simulink model "SYS"  (Simulink 9.2)
settings: Solver=VariableStepAuto  StartTime=0.0  StopTime=10.0  RelTol=1e-3
settings Model: Creator=maman  LastModifiedBy=maman
settings DataIOCC: LimitDataPoints=off  SaveFormat=Dataset  SignalLoggingSaveFormat=Dataset
settings OptimizationCC: LifeSpan=auto
settings DebuggingCC: UnderspecifiedInitializationDetection=Simplified  MergeDetectMultiDrivingBlocksExec=error  FcnCallInpInsideContextMsg=error  StateNameClashWarn=none  SFUnexpectedBacktrackingDiag=error  SFNoUnconditionalDefaultTransitionDiag=error  SFExecutionAtInitializationDiag=warning
settings HardwareCC: ProdBitPerPointer=64  ProdBitPerSizeT=64  ProdBitPerPtrDiffT=64  ProdLargestAtomicFloat=Float  ProdIntDivRoundTo=Zero  ProdEndianess=LittleEndian  ProdWordSize=64  ProdHWDeviceType=Intel->x86-64 (Windows64)
settings ModelReferenceCC: PropagateSignalLabelsOutOfModel=on
settings SFSimCC: SimUseLocalCustomCode=on
settings RTWCC: RTWUseLocalCustomCode=on
settings CodeAppCC: StateflowObjectComments=off
settings GRTTargetCC: TargetLangStandard=C99 (ISO)  GeneratePreprocessorConditionals=Use local settings  CombineOutputUpdateFcns=on  GRTInterface=off
settings ConfigComp: CovMetricSettings=dwe  CovHtmlReporting=off  CovSaveCumulativeToWorkspaceVar=off  CovSaveSingleToWorkspaceVar=off  CovExternalEMLEnable=on

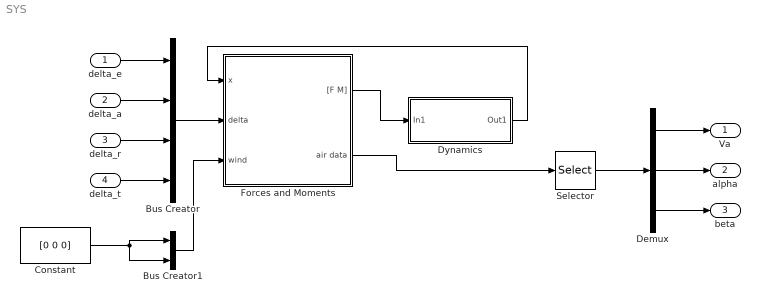
== system SYS ==
  delta_e : Inport
  delta_a : Inport  Port=2
  delta_r : Inport  Port=3
  delta_t : Inport  Port=4
  Bus Creator : BusCreator  Inputs=4
  Bus Creator1 : BusCreator  Inputs=2
  Constant : Constant  Value=[0 0 0]
  Demux : Demux  Outputs=3
  Dynamics : Subsystem  TreatAsAtomicUnit=on
  Forces and Moments : Subsystem  TreatAsAtomicUnit=on
  Selector : Selector  NumberOfDimensions=2  InputPortWidth=3  IndexOptions=Index vector (dialog),Index vector (dialog)  Indices=[1 3],1  OutputSizes=1,1
  Va : Outport
  alpha : Outport  Port=2
  beta : Outport  Port=3
  wires:
  delta_e/1 -> Bus Creator/1
  delta_a/1 -> Bus Creator/2
  delta_r/1 -> Bus Creator/3
  delta_t/1 -> Bus Creator/4
  Bus Creator/1 -> Forces and Moments/2(delta)
  Bus Creator1/1 -> Forces and Moments/3(wind)
  Forces and Moments/1("[F M]") -> Dynamics/1(In1)
  Dynamics/1(Out1) -> Forces and Moments/1(x)
  Forces and Moments/2(air data) -> Selector/1
  Demux/2 -> alpha/1
  Demux/1 -> Va/1
  Demux/3 -> beta/1
  Selector/1 -> Demux/1
  Constant/1 -> Bus Creator1/2, Bus Creator1/1

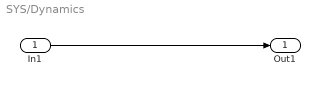
== system SYS/Dynamics ==
  In1 : Inport
  Out1 : Outport
  wires:
  In1/1 -> Out1/1

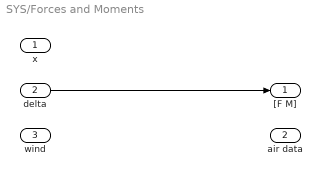
== system SYS/Forces and Moments ==
  x : Inport
  delta : Inport  Port=2
  wind : Inport  Port=3
  "[F M]" : Outport
  air data : Outport  Port=2
  wires:
  delta/1 -> "[F M]"/1
